simulink model "st1"  (R2018b)
settings: Solver=ode45  StartTime=0.0  StopTime=10.0  RelTol=1e-3
settings Model: Creator=12732  LastModifiedBy=12732
settings DataIOCC: SaveFormat=Array

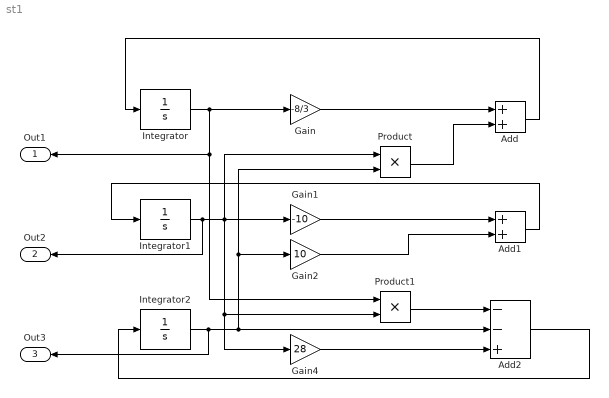
== system st1 ==
  Add : Sum
  Add1 : Sum
  Add2 : Sum  Inputs=--+
  Gain : Gain  Gain=-8/3
  Gain1 : Gain  Gain=-10
  Gain2 : Gain  Gain=10
  Gain4 : Gain  Gain=28
  Integrator : Integrator
  Integrator1 : Integrator
  Integrator2 : Integrator  InitialCondition=10^-10
  Product : Product
  Product1 : Product
  Out1 : Outport
  Out2 : Outport  Port=2
  Out3 : Outport  Port=3
  wires:
  Integrator1/1 -> Out2/1, Product1/2, Gain4/1, Gain1/1, Product/1
  Integrator2/1 -> Out3/1, Gain2/1, Product/2, Add2/2
  Gain/1 -> Add/1
  Product/1 -> Add/2
  Add/1 -> Integrator/1
  Gain1/1 -> Add1/1
  Gain2/1 -> Add1/2
  Add1/1 -> Integrator1/1
  Integrator/1 -> Out1/1, Product1/1, Gain/1
  Gain4/1 -> Add2/3
  Product1/1 -> Add2/1
  Add2/1 -> Integrator2/1
